simulink model "quadcopter_example"  (R2018b)
settings: Solver=VariableStepAuto  StartTime=0.0  StopTime=15  RelTol=1e-3
InitFcn:
  | quadcopter_example_initfcn
values from neighbouring files (symbols this model uses):
  A_osqp = [Aeq; Aineq]    [quadcopter_example_initfcn.m]
  Ad = [1       0       0   0   0   0   0.1     0       0    0       0       0 ... (first row only)    [quadcopter_example_initfcn.m]
  Bd = [0      -0.0726  0       0.0726 ... (first row only)    [quadcopter_example_initfcn.m]
  Cd = eye(nx)    [quadcopter_example_initfcn.m]
  Dd = zeros(nx,nu)    [quadcopter_example_initfcn.m]
  l_osqp = [leq; lineq]    [quadcopter_example_initfcn.m]
  N = 10    [quadcopter_example_initfcn.m]
  P_osqp = blkdiag( kron(speye(N), Q), QN, kron(speye(N), R) )    [quadcopter_example_initfcn.m]
  q_osqp = [repmat(-Q*xr, N, 1); -QN*xr; zeros(N*nu, 1)]    [quadcopter_example_initfcn.m]
  u_osqp = [ueq; uineq]    [quadcopter_example_initfcn.m]
  x0 = zeros(12,1)    [quadcopter_example_initfcn.m]
undefined symbols (not defined in the file or in its folder): nu, nx
libraries: osqp_library x1, simulink x1
settings Model: Creator=pgoulart  LastModifiedBy=pgoulart

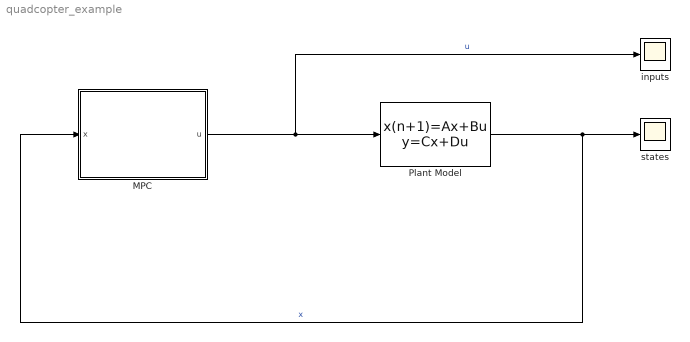
== system quadcopter_example ==
  MPC : Subsystem
  Plant Model : DiscreteStateSpace  A=Ad  B=Bd  C=Cd  D=Dd  InitialCondition=x0
  "inputs " : Scope
  states : Scope
  wires:
  Plant Model/1 -> MPC/1(x), states/1  "x"
  MPC/1(u) -> "inputs "/1, Plant Model/1  "u"

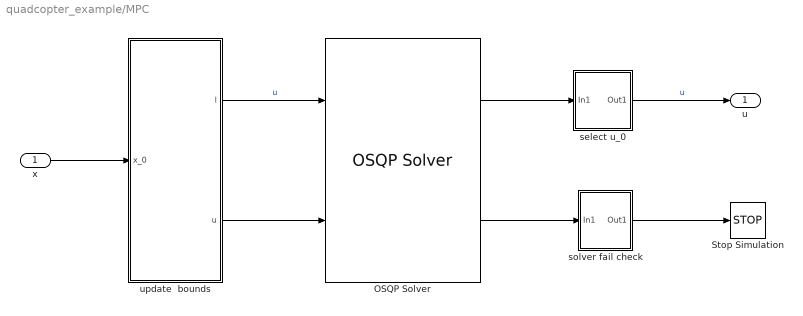
== system quadcopter_example/MPC ==
  x : Inport
  OSQP Solver : osqp_library/OSQP Solver  P=P_osqp  A=A_osqp  q=q_osqp  l=l_osqp  u=u_osqp  opts={'verbose',true }  refactor_style=Never  warmstart_style=Always  has_external_q_input=off  has_external_bound_input=on
  Stop Simulation : Stop
  select u_0 : Subsystem
  solver fail check : Subsystem
  update  bounds : Subsystem
  u : Outport
  wires:
  x/1 -> update  bounds/1(x_0)
  select u_0/1(Out1) -> u/1  "u"
  OSQP Solver/1 -> select u_0/1(In1)
  OSQP Solver/2 -> solver fail check/1(In1)
  solver fail check/1(Out1) -> Stop Simulation/1
  update  bounds/1(l) -> OSQP Solver/1  "u"
  update  bounds/2(u) -> OSQP Solver/2

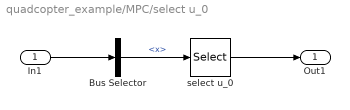
== system quadcopter_example/MPC/select u_0 ==
  In1 : Inport
  Bus Selector : BusSelector  OutputSignals=x
  "select u_0 " : Selector  InputPortWidth=length(q_osqp)  IndexOptions=Index vector (dialog)  Indices=((N+1)*nx+1:(N+1)*nx+nu)  OutputSizes=1
  Out1 : Outport
  wires:
  "select u_0 "/1 -> Out1/1
  In1/1 -> Bus Selector/1
  Bus Selector/1 -> "select u_0 "/1  "<x>"

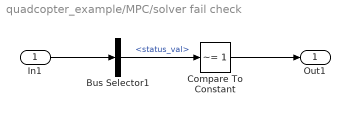
== system quadcopter_example/MPC/solver fail check ==
  In1 : Inport
  Bus Selector1 : BusSelector  OutputSignals=status_val
  Compare To Constant : simulink/Logic and Bit Operations/Compare To Constant  relop=~=  const=1  OutDataTypeStr=boolean
  Out1 : Outport
  wires:
  In1/1 -> Bus Selector1/1
  Compare To Constant/1 -> Out1/1
  Bus Selector1/1 -> Compare To Constant/1  "<status_val>"

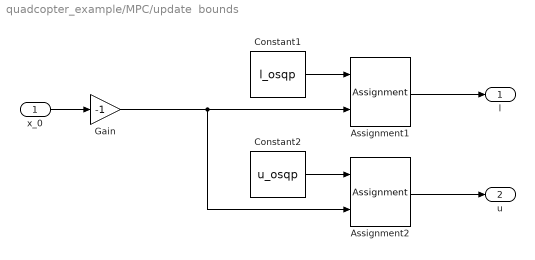
== system quadcopter_example/MPC/update  bounds ==
  x_0 : Inport
  Assignment1 : Assignment  DiagnosticForDimensions=Warning  IndexOptions=Index vector (dialog)  Indices=1:nx  OutputSizes=1
  Assignment2 : Assignment  DiagnosticForDimensions=Warning  IndexOptions=Index vector (dialog)  Indices=1:nx  OutputSizes=1
  Constant1 : Constant  Value=l_osqp
  Constant2 : Constant  Value=u_osqp
  Gain : Gain  Gain=-1
  l : Outport
  u : Outport  Port=2
  wires:
  Assignment1/1 -> l/1
  Constant1/1 -> Assignment1/1
  x_0/1 -> Gain/1
  Assignment2/1 -> u/1
  Gain/1 -> Assignment2/2, Assignment1/2
  Constant2/1 -> Assignment2/1
